simulink model "TestDyn_4CIGs_OP_7"  (R2024b)
settings: Solver=ode1  StartTime=0.0  StopTime=sim_config.Tsim  RelTol=1e-3
undefined symbols (not defined in the file): sim_config
libraries: myLibrary x15, spsThreePhaseVIMeasurementLib x8, spsPower3phInstantaneousLib x6, spspowerguiLib x1
settings Model: Creator=Francesca  LastModifiedBy=Francesca

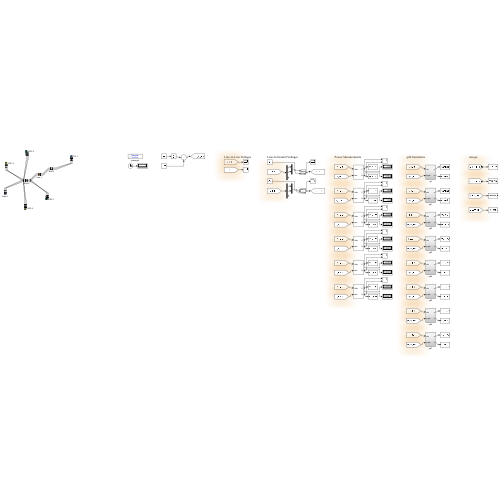
[thumbnail: Simulink's stored preview of the top-level diagram]
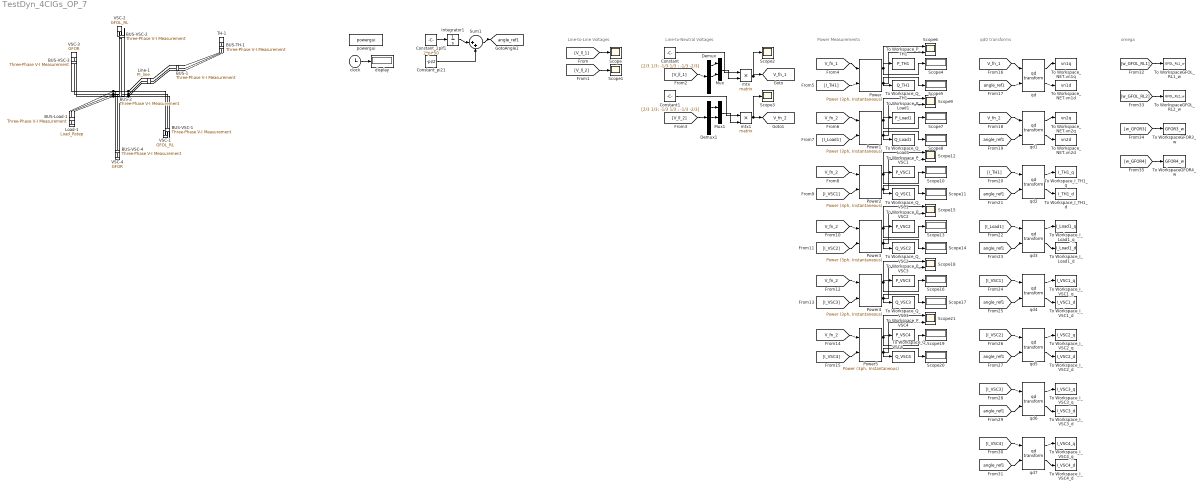
== system TestDyn_4CIGs_OP_7 ==
  note: Line-to-Line Voltages
  note: Line-to-Neutral Voltages
  note: Power Measurements
  note: qd0 transforms
  note: omega
  BUS-1 : spsThreePhaseVIMeasurementLib/Three-Phase V-I Measurement  VoltageMeasurement=phase-to-phase  SetLabelV=on  LabelV=V_ll_1  Vpu=off  VpuLL=off  CurrentMeasurement=yes  SetLabelI=on  LabelI=I_1  Ipu=off  Pbase=100e6  Vbase=500e3  OutputType=Complex  PhasorSimulation=off  PSBequivalent=0
  BUS-2 : spsThreePhaseVIMeasurementLib/Three-Phase V-I Measurement  VoltageMeasurement=phase-to-phase  SetLabelV=on  LabelV=V_ll_2  Vpu=off  VpuLL=off  CurrentMeasurement=yes  SetLabelI=on  LabelI=I_2  Ipu=off  Pbase=100e6  Vbase=500e3  OutputType=Complex  PhasorSimulation=off  PSBequivalent=0
  BUS-Load-1 : spsThreePhaseVIMeasurementLib/Three-Phase V-I Measurement  VoltageMeasurement=phase-to-phase  SetLabelV=on  LabelV=V_Load_1  Vpu=off  VpuLL=off  CurrentMeasurement=yes  SetLabelI=on  LabelI=I_Load1  Ipu=off  Pbase=100e6  Vbase=500e3  OutputType=Complex  PhasorSimulation=off  PSBequivalent=0
  BUS-TH-1 : spsThreePhaseVIMeasurementLib/Three-Phase V-I Measurement  VoltageMeasurement=phase-to-phase  SetLabelV=on  LabelV=V_TH_1  Vpu=off  VpuLL=off  CurrentMeasurement=yes  SetLabelI=on  LabelI=I_TH1  Ipu=off  Pbase=100e6  Vbase=500e3  OutputType=Complex  PhasorSimulation=off  PSBequivalent=0
  BUS-VSC-1 : spsThreePhaseVIMeasurementLib/Three-Phase V-I Measurement  VoltageMeasurement=phase-to-phase  SetLabelV=on  LabelV=V_VSC_1  Vpu=off  VpuLL=off  CurrentMeasurement=yes  SetLabelI=on  LabelI=I_VSC1  Ipu=off  Pbase=100e6  Vbase=500e3  OutputType=Complex  PhasorSimulation=off  PSBequivalent=0
  BUS-VSC-2 : spsThreePhaseVIMeasurementLib/Three-Phase V-I Measurement  VoltageMeasurement=phase-to-phase  SetLabelV=on  LabelV=V_VSC_2  Vpu=off  VpuLL=off  CurrentMeasurement=yes  SetLabelI=on  LabelI=I_VSC2  Ipu=off  Pbase=100e6  Vbase=500e3  OutputType=Complex  PhasorSimulation=off  PSBequivalent=0
  BUS-VSC-3 : spsThreePhaseVIMeasurementLib/Three-Phase V-I Measurement  VoltageMeasurement=phase-to-phase  SetLabelV=on  LabelV=V_VSC_3  Vpu=off  VpuLL=off  CurrentMeasurement=yes  SetLabelI=on  LabelI=I_VSC3  Ipu=off  Pbase=100e6  Vbase=500e3  OutputType=Complex  PhasorSimulation=off  PSBequivalent=0
  BUS-VSC-4 : spsThreePhaseVIMeasurementLib/Three-Phase V-I Measurement  VoltageMeasurement=phase-to-phase  SetLabelV=on  LabelV=V_VSC_4  Vpu=off  VpuLL=off  CurrentMeasurement=yes  SetLabelI=on  LabelI=I_VSC4  Ipu=off  Pbase=100e6  Vbase=500e3  OutputType=Complex  PhasorSimulation=off  PSBequivalent=0
  Constant : Constant  Value=[2/3 1/3; -1/3 1/3 ; -1/3 -2/3]
  Constant1 : Constant  Value=[2/3 1/3; -1/3 1/3 ; -1/3 -2/3]
  Constant_2pif1 : Constant  Value=2*pi*50
  Constant_pi21 : Constant  Value=-pi/2
  Demux : Demux  Outputs=3
  Demux1 : Demux  Outputs=3
  Integrator1 : Integrator
  Line-1 : myLibrary/PI_line  T_line_global=T_NET  initLine_global=init_line  num=1  set_C0=ones(1,6)  set_iL0=0
  Load-1 : myLibrary/Load_Rstep  T_load_global=T_load  initLoad_global=init_load  num=1  tstep=sim_config.tstep  Radd=Rload_add
  Mux : Mux  Inputs=2
  Mux1 : Mux  Inputs=2
  Power{,1..5} (6 alike) : spsPower3phInstantaneousLib/Power (3ph, Instantaneous)
  Scope{,1..3} (4 alike) : Scope
  Scope{4..5,7..8,10..11,13..14,16..17,19..20} (12 alike) : Display
  Scope{6,9,12,15,18,21} (6 alike) : Scope  NumInputPorts=2
  Sum1 : Sum  Inputs=|++
  TH-1 : myLibrary/TH  T_TH_global=T_TH  initTH_global=init_TH  num=1
  To WorkspaceGFOL_RL1_w : ToWorkspace  VariableName=GFOL_RL1_w  SampleTime=sim_config.Tsample
  To WorkspaceGFOL_RL2_w : ToWorkspace  VariableName=GFOL_RL2_w  SampleTime=sim_config.Tsample
  To WorkspaceGFOR3_w : ToWorkspace  VariableName=GFOR3_w  SampleTime=sim_config.Tsample
  To WorkspaceGFOR4_w : ToWorkspace  VariableName=GFOR4_w  SampleTime=sim_config.Tsample
  To Workspace_I_Load1_d : ToWorkspace  VariableName=I_Load1_d  SampleTime=sim_config.Tsample
  To Workspace_I_Load1_q : ToWorkspace  VariableName=I_Load1_q  SampleTime=sim_config.Tsample
  To Workspace_I_TH1_d : ToWorkspace  VariableName=I_TH1_d  SampleTime=sim_config.Tsample
  To Workspace_I_TH1_q : ToWorkspace  VariableName=I_TH1_q  SampleTime=sim_config.Tsample
  To Workspace_I_VSC1_d : ToWorkspace  VariableName=I_VSC1_d  SampleTime=sim_config.Tsample
  To Workspace_I_VSC1_q : ToWorkspace  VariableName=I_VSC1_q  SampleTime=sim_config.Tsample
  To Workspace_I_VSC2_d : ToWorkspace  VariableName=I_VSC2_d  SampleTime=sim_config.Tsample
  To Workspace_I_VSC2_q : ToWorkspace  VariableName=I_VSC2_q  SampleTime=sim_config.Tsample
  To Workspace_I_VSC3_d : ToWorkspace  VariableName=I_VSC3_d  SampleTime=sim_config.Tsample
  To Workspace_I_VSC3_q : ToWorkspace  VariableName=I_VSC3_q  SampleTime=sim_config.Tsample
  To Workspace_I_VSC4_d : ToWorkspace  VariableName=I_VSC4_d  SampleTime=sim_config.Tsample
  To Workspace_I_VSC4_q : ToWorkspace  VariableName=I_VSC4_q  SampleTime=sim_config.Tsample
  To Workspace_NET.vn1d : ToWorkspace  VariableName=vn1d  SampleTime=sim_config.Tsample
  To Workspace_NET.vn1q : ToWorkspace  VariableName=vn1q  SampleTime=sim_config.Tsample
  To Workspace_NET.vn2d : ToWorkspace  VariableName=vn2d  SampleTime=sim_config.Tsample
  To Workspace_NET.vn2q : ToWorkspace  VariableName=vn2q  SampleTime=sim_config.Tsample
  To Workspace_P_Load1 : ToWorkspace  VariableName=P_Load1  SampleTime=sim_config.Tsample
  To Workspace_P_TH1 : ToWorkspace  VariableName=P_TH1  SampleTime=sim_config.Tsample
  To Workspace_P_VSC1 : ToWorkspace  VariableName=P_VSC1  SampleTime=sim_config.Tsample
  To Workspace_P_VSC2 : ToWorkspace  VariableName=P_VSC2  SampleTime=sim_config.Tsample
  To Workspace_P_VSC3 : ToWorkspace  VariableName=P_VSC3  SampleTime=sim_config.Tsample
  To Workspace_P_VSC4 : ToWorkspace  VariableName=P_VSC4  SampleTime=sim_config.Tsample
  To Workspace_Q_Load1 : ToWorkspace  VariableName=Q_Load1  SampleTime=sim_config.Tsample
  To Workspace_Q_TH1 : ToWorkspace  VariableName=Q_TH1  SampleTime=sim_config.Tsample
  To Workspace_Q_VSC1 : ToWorkspace  VariableName=Q_VSC1  SampleTime=sim_config.Tsample
  To Workspace_Q_VSC2 : ToWorkspace  VariableName=Q_VSC2  SampleTime=sim_config.Tsample
  To Workspace_Q_VSC3 : ToWorkspace  VariableName=Q_VSC3  SampleTime=sim_config.Tsample
  To Workspace_Q_VSC4 : ToWorkspace  VariableName=Q_VSC4  SampleTime=sim_config.Tsample
  VSC-1 : myLibrary/GFOL_RL  T_VSC_global=T_VSC  initVSC_global=init_VSC  num=1
  VSC-2 : myLibrary/GFOL_RL  T_VSC_global=T_VSC  initVSC_global=init_VSC  num=2
  VSC-3 : myLibrary/GFOR  T_VSC_global=T_VSC  initVSC_global=init_VSC  num=3
  VSC-4 : myLibrary/GFOR  T_VSC_global=T_VSC  initVSC_global=init_VSC  num=4
  clock : Clock
  display : Display
  mtx : Product  Multiplication=Matrix(*)
  mtx1 : Product  Multiplication=Matrix(*)
  powergui : spspowerguiLib/powergui  Priority=1  SimulationMode=Discrete  SampleTime=sim_config.Ts  frequency=60  Iterations=50  frequencyindice=50  Pbase=100e6  ErrMax=1e-4  UnitsV=kV  UnitsW=MW  buscounter=0  FunctionMessages=off  echomessages=off  EnableUseOfTLC=off  CurrentSourceSwitches=off  DisableSnubberDevices=off  DisableRonSwitches=off  DisableVfSwitches=off  DisplayEquations=off  AutomaticDiscreteSolvers=off  SolverType=Tustin/Backward Euler (TBE)  Interpol=off  ExternalGateDelay=off  methode=off  Ts=100  x0status=blocks  SPID=on  SwTol=0  HookPort=off  NonlinearTolerance=1e-4  nMaxIteration=100  ContinueOnMaxIteration=off  RestoreLinks=warning  ResistiveCurrentMeasurement=off  Frange=[0:2:500]  Ylog=off  Xlog=on  ShowGrid=off  save=off  variable=ZData  structure=0  ZoomFFT=off  StartTime=0.0  cycles=1  DisplayStyle=1  fundamental=60  FreqAxis=off  MaxFrequency=1000  frequencyindicesteady=1  RmsSteady=1  display=off
  qd{,1..7} (8 alike) : myLibrary/qd transform  SystemSampleTime=-1  VariantActivationTime=update diagram  AllowFlexibleInterface=on  Latency=0  AutoFrameSizeCalculation=off
  tag scope: V_fn_1=global, V_fn_2=global, angle_ref1=global
  wires:
  clock/1 -> display/1
  Constant_2pif1/1 -> Integrator1/1
  Integrator1/1 -> Sum1/1
  Constant_pi21/1 -> Sum1/2
  Sum1/1 -> [angle_ref1]
  [V_ll_1] -> Scope/1
  [V_ll_2] -> Scope1/1
  [V_ll_1] -> Demux/1
  Demux/1 -> Mux/1
  Demux/2 -> Mux/2
  Mux/1 -> mtx/2
  Constant/1 -> mtx/1
  mtx/1 -> [V_fn_1], Scope2/1
  [V_ll_2] -> Demux1/1
  Demux1/1 -> Mux1/1
  Demux1/2 -> Mux1/2
  Mux1/1 -> mtx1/2
  Constant1/1 -> mtx1/1
  mtx1/1 -> [V_fn_2], Scope3/1
  [V_fn_1] -> Power/1
  [I_TH1] -> Power/2
  Power/1 -> To Workspace_P_TH1/1, Scope4/1, Scope6/1
  Power/2 -> To Workspace_Q_TH1/1, Scope5/1, Scope6/2
  [V_fn_2] -> Power1/1
  [I_Load1] -> Power1/2
  Power1/1 -> To Workspace_P_Load1/1, Scope7/1, Scope9/1
  Power1/2 -> To Workspace_Q_Load1/1, Scope8/1, Scope9/2
  [V_fn_2] -> Power2/1
  [I_VSC1] -> Power2/2
  Power2/1 -> To Workspace_P_VSC1/1, Scope10/1, Scope12/1
  Power2/2 -> To Workspace_Q_VSC1/1, Scope11/1, Scope12/2
  [V_fn_2] -> Power3/1
  [I_VSC2] -> Power3/2
  Power3/1 -> To Workspace_P_VSC2/1, Scope13/1, Scope15/1
  Power3/2 -> To Workspace_Q_VSC2/1, Scope14/1, Scope15/2
  [V_fn_2] -> Power4/1
  [I_VSC3] -> Power4/2
  Power4/1 -> To Workspace_P_VSC3/1, Scope16/1, Scope18/1
  Power4/2 -> To Workspace_Q_VSC3/1, Scope17/1, Scope18/2
  [V_fn_2] -> Power5/1
  [I_VSC4] -> Power5/2
  Power5/1 -> To Workspace_P_VSC4/1, Scope19/1, Scope21/1
  Power5/2 -> To Workspace_Q_VSC4/1, Scope20/1, Scope21/2
  [V_fn_1] -> qd/1
  [angle_ref1] -> qd/2
  qd/1 -> To Workspace_NET.vn1q/1
  qd/2 -> To Workspace_NET.vn1d/1
  [V_fn_2] -> qd1/1
  [angle_ref1] -> qd1/2
  qd1/1 -> To Workspace_NET.vn2q/1
  qd1/2 -> To Workspace_NET.vn2d/1
  [I_TH1] -> qd2/1
  [angle_ref1] -> qd2/2
  qd2/1 -> To Workspace_I_TH1_q/1
  qd2/2 -> To Workspace_I_TH1_d/1
  [I_Load1] -> qd3/1
  [angle_ref1] -> qd3/2
  qd3/1 -> To Workspace_I_Load1_q/1
  qd3/2 -> To Workspace_I_Load1_d/1
  [I_VSC1] -> qd4/1
  [angle_ref1] -> qd4/2
  qd4/1 -> To Workspace_I_VSC1_q/1
  qd4/2 -> To Workspace_I_VSC1_d/1
  [I_VSC2] -> qd5/1
  [angle_ref1] -> qd5/2
  qd5/1 -> To Workspace_I_VSC2_q/1
  qd5/2 -> To Workspace_I_VSC2_d/1
  [I_VSC3] -> qd6/1
  [angle_ref1] -> qd6/2
  qd6/1 -> To Workspace_I_VSC3_q/1
  qd6/2 -> To Workspace_I_VSC3_d/1
  [I_VSC4] -> qd7/1
  [angle_ref1] -> qd7/2
  qd7/1 -> To Workspace_I_VSC4_q/1
  qd7/2 -> To Workspace_I_VSC4_d/1
  [w_GFOL_RL1] -> To WorkspaceGFOL_RL1_w/1
  [w_GFOL_RL2] -> To WorkspaceGFOL_RL2_w/1
  [w_GFOR3] -> To WorkspaceGFOR3_w/1
  [w_GFOR4] -> To WorkspaceGFOR4_w/1
  connections:
  BUS-1/RConn1 -- BUS-TH-1/RConn1
  BUS-1/RConn2 -- BUS-TH-1/RConn2
  BUS-1/RConn3 -- BUS-TH-1/RConn3
  BUS-TH-1/LConn1 -- TH-1/RConn1
  BUS-TH-1/LConn2 -- TH-1/RConn2
  BUS-TH-1/LConn3 -- TH-1/RConn3
  BUS-1/LConn1 -- Line-1/LConn1
  BUS-1/LConn2 -- Line-1/LConn2
  BUS-1/LConn3 -- Line-1/LConn3
  BUS-2/RConn1 -- Line-1/RConn1 -- BUS-VSC-1/RConn1
  BUS-2/RConn2 -- Line-1/RConn2 -- BUS-VSC-1/RConn2
  BUS-2/RConn3 -- Line-1/RConn3 -- BUS-VSC-1/RConn3
  BUS-Load-1/LConn1 -- BUS-2/LConn1 -- BUS-VSC-2/RConn1 -- BUS-VSC-3/RConn1 -- BUS-VSC-4/RConn1
  BUS-Load-1/LConn2 -- BUS-2/LConn2 -- BUS-VSC-2/RConn2 -- BUS-VSC-3/RConn2 -- BUS-VSC-4/RConn2
  BUS-Load-1/LConn3 -- BUS-2/LConn3 -- BUS-VSC-2/RConn3 -- BUS-VSC-3/RConn3 -- BUS-VSC-4/RConn3
  BUS-Load-1/RConn1 -- Load-1/LConn1
  BUS-Load-1/RConn2 -- Load-1/LConn2
  BUS-Load-1/RConn3 -- Load-1/LConn3
  BUS-VSC-1/LConn1 -- VSC-1/RConn1
  BUS-VSC-1/LConn2 -- VSC-1/RConn2
  BUS-VSC-1/LConn3 -- VSC-1/RConn3
  BUS-VSC-2/LConn1 -- VSC-2/RConn1
  BUS-VSC-2/LConn2 -- VSC-2/RConn2
  BUS-VSC-2/LConn3 -- VSC-2/RConn3
  BUS-VSC-3/LConn1 -- VSC-3/RConn1
  BUS-VSC-3/LConn2 -- VSC-3/RConn2
  BUS-VSC-3/LConn3 -- VSC-3/RConn3
  BUS-VSC-4/LConn1 -- VSC-4/RConn1
  BUS-VSC-4/LConn2 -- VSC-4/RConn2
  BUS-VSC-4/LConn3 -- VSC-4/RConn3
